simulink model "NewOrbitSimulation"  (R2015a)
settings: Solver=ode45  StartTime=0.0  StopTime=1000  FixedStep=.1  RelTol=1e-9
InitFcn:
  | PlanetSelect;
StopFcn:
  | TotalDeltaV
undefined symbols (not defined in the file or in its folder): AtmoAlt_planet, AtmoData, Cd, CraftInitialP, CraftInitialV, DragData, g0, GM_planet, GndAlt_planet, LastStage, Omega_planet, PitchOverAlt, PitchOverAngle, PitchSwitch, R_planet, RefSurfArea, SSIGN, TargetOrbit, Throttle
libraries: simulink_extras x6, dspmathops x5, simulink x3, vrlib x2
settings Model: PauseTimes=122  SnapshotInterval=1  Creator=raulm_000  LastModifiedBy=raulm_000
settings DataIOCC: ExternalInput=[Throttle,SSIGN]  LimitDataPoints=off  SaveFinalState=on

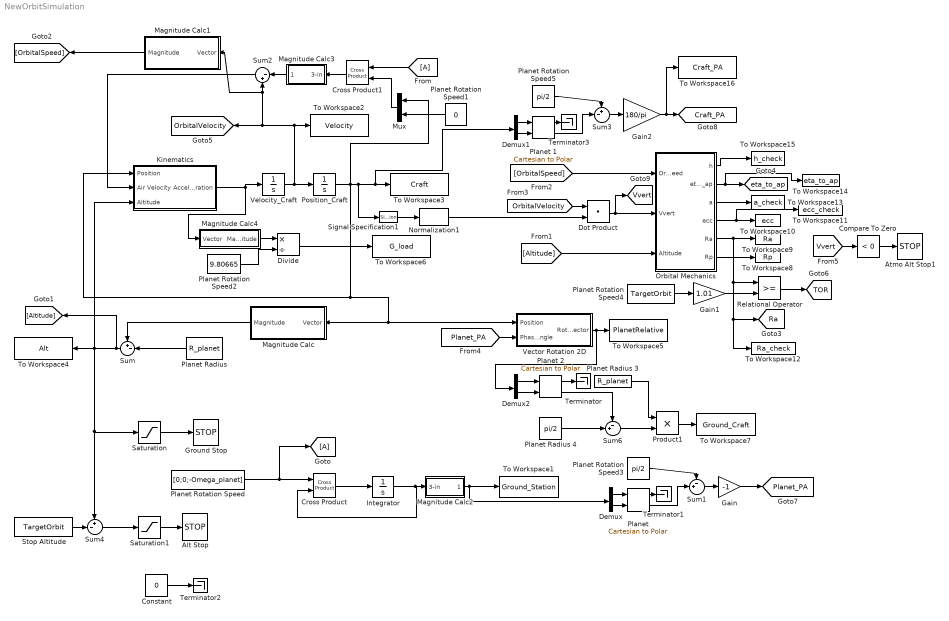
== system NewOrbitSimulation ==
  " Alt Stop" : Stop
  Atmo Alt Stop1 : Stop
  Compare To Zero : simulink/Logic and Bit Operations/Compare To Zero  relop=<  OutDataTypeStr=boolean
  Constant : Constant  Value=0
  Cross Product : vrlib/Utilities/Cross Product
  Cross Product1 : vrlib/Utilities/Cross Product
  Demux : Demux  Outputs=2
  Demux1 : Demux  Outputs=2
  Demux2 : Demux  Outputs=2
  Divide : Product  Inputs=*/
  Dot Product : DotProduct  InputSameDT=on  OutDataTypeStr=Inherit: Inherit via internal rule
  Gain : Gain  Gain=-1
  Gain1 : Gain  Gain=1.01
  Gain2 : Gain  Gain=180/pi
  Ground Stop : Stop
  Integrator : Integrator  InitialCondition=[0;R_planet;0]
  Kinematics : Subsystem
  Magnitude Calc : Subsystem
  Magnitude Calc1 : Subsystem
  Magnitude Calc2 : Subsystem
  Magnitude Calc3 : Subsystem
  Magnitude Calc4 : Subsystem
  Mux : Mux  Inputs=2
  Normalization1 : dspmathops/Normalization  NormType=2-norm  Bias=1e-10  NormOver=Specified dimension  ColComp=off  Dimension=1  outputMin=[]  outputMax=[]  accumDataTypeStr=Inherit: Same as product output  accumLastDataTypeStr=Inherit: Same as product output  roundingMode=Floor  overflowMode=off
  Orbital Mechanics : MATLAB Function  TreatAsAtomicUnit=on
  "Planet " : simulink_extras/Transformations/Cartesian to Polar
  Planet 1 : simulink_extras/Transformations/Cartesian to Polar
  Planet 2 : simulink_extras/Transformations/Cartesian to Polar
  "Planet Radius " : Constant  Value=R_planet
  Planet Radius 3 : Constant  Value=R_planet
  Planet Radius 4 : Constant  Value=pi/2
  Planet Rotation Speed : Constant  Value=[0;0;-Omega_planet]
  Planet Rotation Speed1 : Constant  Value=0
  Planet Rotation Speed2 : Constant  Value=9.80665
  Planet Rotation Speed3 : Constant  Value=pi/2
  Planet Rotation Speed4 : Constant  Value=TargetOrbit
  Planet Rotation Speed5 : Constant  Value=pi/2
  Position_Craft : Integrator  InitialCondition=CraftInitialP
  Product1 : Product
  Relational Operator : RelationalOperator  OutDataTypeStr=boolean
  Saturation : Saturate  UpperLimit=0
  Saturation1 : Saturate  UpperLimit=1  LowerLimit=0
  Signal Specification1 : SignalSpecification  Dimensions=2
  Stop Altitude : Constant  Value=TargetOrbit
  Sum : Sum  Inputs=+-|
  Sum1 : Sum  Inputs=-+|
  Sum2 : Sum  Inputs=|-+
  Sum3 : Sum  Inputs=+-|
  Sum4 : Sum  Inputs=+-|
  Sum6 : Sum  Inputs=-+|
  Terminator{,1..3} (4 alike) : Terminator
  To Workspace1 : ToWorkspace  VariableName=Ground_Station  SampleTime=-1
  To Workspace10 : ToWorkspace  VariableName=ecc  SampleTime=-1
  To Workspace11 : ToWorkspace  VariableName=ecc_check  SampleTime=-1
      settings: MaxDataPoints=1
  To Workspace12 : ToWorkspace  VariableName=Ra_check  SampleTime=-1
      settings: MaxDataPoints=1
  To Workspace13 : ToWorkspace  VariableName=a_check  SampleTime=-1
      settings: MaxDataPoints=1
  To Workspace14 : ToWorkspace  VariableName=eta_to_ap  SampleTime=-1
  To Workspace15 : ToWorkspace  VariableName=h_check  SampleTime=-1
      settings: MaxDataPoints=1
  To Workspace16 : ToWorkspace  VariableName=Craft_PA  SampleTime=-1
  To Workspace2 : ToWorkspace  VariableName=Velocity  SampleTime=-1
  To Workspace3 : ToWorkspace  VariableName=Craft  SampleTime=-1
  To Workspace4 : ToWorkspace  VariableName=Alt  SampleTime=-1
  To Workspace5 : ToWorkspace  VariableName=PlanetRelative  SampleTime=-1
  To Workspace6 : ToWorkspace  VariableName=G_load  SampleTime=-1
  To Workspace7 : ToWorkspace  VariableName=Ground_Craft  SampleTime=-1
  To Workspace8 : ToWorkspace  VariableName=Rp  SampleTime=-1
  To Workspace9 : ToWorkspace  VariableName=Ra  SampleTime=-1
  Vector Rotation 2D : Subsystem
  Velocity_Craft : Integrator  InitialCondition=CraftInitialV-[.1;0]
  tag scope: Craft_PA=global, OrbitalVelocity=global, Planet_PA=global, Ra=global, TOR=global, Vvert=global, eta_to_ap=global
  wires:
  Planet Rotation Speed/1 -> [A], Cross Product/1
  Integrator/1 -> Cross Product/2, Magnitude Calc2/1(3-in)
  Cross Product/1 -> Integrator/1
  Velocity_Craft/1 -> Position_Craft/1, [OrbitalVelocity], Magnitude Calc1/1(Vector), Sum2/2, To Workspace2/1
  Position_Craft/1 -> Mux/1, Kinematics/1(Position), Vector Rotation 2D/1(Position), Magnitude Calc/1(Vector), Signal Specification1/1, Demux1/1, To Workspace3/1
  Magnitude Calc/1("Magnitude ") -> Sum/1
  "Planet Radius "/1 -> Sum/2
  Sum/1 -> [Altitude], Kinematics/3("Altitude "), Sum4/1, Saturation/1, To Workspace4/1
  Magnitude Calc2/1("2-out ") -> Demux/1, To Workspace1/1
  Sum2/1 -> Kinematics/2(Air Velocity)
  Kinematics/1("Acceleration ") -> Velocity_Craft/1, Magnitude Calc4/1(Vector)
  Saturation/1 -> Ground Stop/1
  [A] -> Cross Product1/1
  Cross Product1/1 -> Magnitude Calc3/1(3-in)
  Mux/1 -> Cross Product1/2
  Planet Rotation Speed1/1 -> Mux/2
  Magnitude Calc3/1("2-out ") -> Sum2/1
  Stop Altitude/1 -> Sum4/2
  Sum4/1 -> Saturation1/1
  Magnitude Calc4/1("Magnitude ") -> Divide/1
  Planet Rotation Speed2/1 -> Divide/2
  Divide/1 -> To Workspace6/1
  Demux/1 -> "Planet "/1
  Demux/2 -> "Planet "/2
  Vector Rotation 2D/1("Rotated Vector ") -> Demux2/1, To Workspace5/1
  "Planet "/2 -> Sum1/2
  Planet Rotation Speed3/1 -> Sum1/1
  Sum1/1 -> Gain/1
  Planet 2/2 -> Sum6/1
  Planet Radius 3/1 -> Product1/1
  Product1/1 -> To Workspace7/1
  Planet Radius 4/1 -> Sum6/2
  Sum6/1 -> Product1/2
  Demux2/1 -> Planet 2/1
  Demux2/2 -> Planet 2/2
  Orbital Mechanics/5(Ra) -> To Workspace12/1, [Ra], Relational Operator/1, To Workspace9/1
  Orbital Mechanics/6(Rp) -> To Workspace8/1
  Orbital Mechanics/4(ecc) -> To Workspace11/1, To Workspace10/1
  Planet Rotation Speed4/1 -> Gain1/1
  Magnitude Calc1/1("Magnitude ") -> [OrbitalSpeed]
  [Altitude] -> Orbital Mechanics/3(Altitude)
  [OrbitalSpeed] -> Orbital Mechanics/1(OrbitalSpeed)
  Relational Operator/1 -> [TOR]
  Planet 2/1 -> Terminator/1
  "Planet "/1 -> Terminator1/1
  Orbital Mechanics/3(a) -> To Workspace13/1
  Orbital Mechanics/2(eta_to_ap) -> To Workspace14/1, [eta_to_ap]
  Orbital Mechanics/1(h) -> To Workspace15/1
  Signal Specification1/1 -> Normalization1/1
  Normalization1/1 -> Dot Product/2
  [OrbitalVelocity] -> Dot Product/1
  Dot Product/1 -> Orbital Mechanics/2(Vvert), [Vvert]
  Gain/1 -> [Planet_PA]
  [Planet_PA] -> Vector Rotation 2D/2(Phase Angle)
  Demux1/1 -> Planet 1/1
  Demux1/2 -> Planet 1/2
  Planet 1/2 -> Sum3/2
  Planet Rotation Speed5/1 -> Sum3/1
  Planet 1/1 -> Terminator3/1
  Constant/1 -> Terminator2/1
  Saturation1/1 -> " Alt Stop"/1
  Gain1/1 -> Relational Operator/2
  [Vvert] -> Compare To Zero/1
  Compare To Zero/1 -> Atmo Alt Stop1/1
  Sum3/1 -> Gain2/1
  Gain2/1 -> To Workspace16/1, [Craft_PA]

== system NewOrbitSimulation/Kinematics ==
  Position : Inport
  Air Velocity : Inport  Port=2
  "Altitude " : Inport  Port=3
  Aerodynamics : Subsystem
  Gravitational Acceleration : Subsystem
  Sum3 : Sum  Inputs=+++
  Thrust : Subsystem
  "Acceleration " : Outport
  wires:
  Position/1 -> Thrust/2(Position), Gravitational Acceleration/1(Position)
  Air Velocity/1 -> Thrust/3(AirVelocity), Aerodynamics/1(Air Velocity)
  "Altitude "/1 -> Thrust/1(Altitude), Aerodynamics/2("Altitude ")
  Aerodynamics/1("Aeroaccel ") -> Sum3/2
  Gravitational Acceleration/1("Gavity ") -> Sum3/1
  Sum3/1 -> "Acceleration "/1
  Thrust/1("ThrustAccel ") -> Sum3/3

== system NewOrbitSimulation/Magnitude Calc ==
  Vector : Inport
  Add : Sum
  Demux : Demux  Outputs=2
  Math Function : Math  Operator=square  SaturateOnIntegerOverflow=on
  Math Function1 : Math  Operator=square  SaturateOnIntegerOverflow=on
  Sqrt : Sqrt  SaturateOnIntegerOverflow=on
  "Magnitude " : Outport
  wires:
  Demux/1 -> Math Function1/1
  Demux/2 -> Math Function/1
  Math Function/1 -> Add/2
  Add/1 -> Sqrt/1
  Vector/1 -> Demux/1
  Math Function1/1 -> Add/1
  Sqrt/1 -> "Magnitude "/1

== system NewOrbitSimulation/Magnitude Calc1 ==
  Vector : Inport
  Add : Sum
  Demux : Demux  Outputs=2
  Math Function : Math  Operator=square  SaturateOnIntegerOverflow=on
  Math Function1 : Math  Operator=square  SaturateOnIntegerOverflow=on
  Sqrt : Sqrt  SaturateOnIntegerOverflow=on
  "Magnitude " : Outport
  wires:
  Demux/1 -> Math Function1/1
  Demux/2 -> Math Function/1
  Math Function/1 -> Add/2
  Add/1 -> Sqrt/1
  Vector/1 -> Demux/1
  Math Function1/1 -> Add/1
  Sqrt/1 -> "Magnitude "/1

== system NewOrbitSimulation/Magnitude Calc2 ==
  3-in : Inport
  Demux4 : Demux  Outputs=3
  Mux2 : Mux  Inputs=2
  Terminator3 : Terminator
  "2-out " : Outport
  wires:
  3-in/1 -> Demux4/1
  Demux4/3 -> Terminator3/1
  Demux4/1 -> Mux2/1
  Demux4/2 -> Mux2/2
  Mux2/1 -> "2-out "/1

== system NewOrbitSimulation/Magnitude Calc3 ==
  3-in : Inport
  Demux4 : Demux  Outputs=3
  Mux2 : Mux  Inputs=2
  Terminator3 : Terminator
  "2-out " : Outport
  wires:
  3-in/1 -> Demux4/1
  Demux4/3 -> Terminator3/1
  Demux4/1 -> Mux2/1
  Demux4/2 -> Mux2/2
  Mux2/1 -> "2-out "/1

== system NewOrbitSimulation/Magnitude Calc4 ==
  Vector : Inport
  Add : Sum
  Demux : Demux  Outputs=2
  Math Function : Math  Operator=square  SaturateOnIntegerOverflow=on
  Math Function1 : Math  Operator=square  SaturateOnIntegerOverflow=on
  Sqrt : Sqrt  SaturateOnIntegerOverflow=on
  "Magnitude " : Outport
  wires:
  Demux/1 -> Math Function1/1
  Demux/2 -> Math Function/1
  Math Function/1 -> Add/2
  Add/1 -> Sqrt/1
  Vector/1 -> Demux/1
  Math Function1/1 -> Add/1
  Sqrt/1 -> "Magnitude "/1

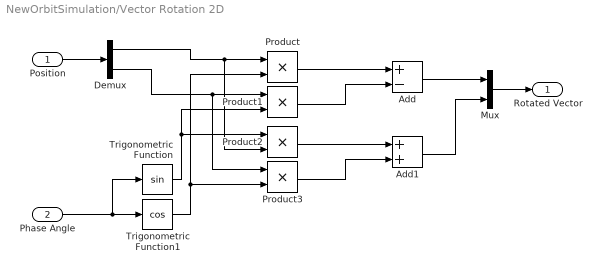
== system NewOrbitSimulation/Vector Rotation 2D ==
  Position : Inport
  Phase Angle : Inport  Port=2
  Add : Sum  Inputs=+-
  Add1 : Sum
  Demux : Demux  Outputs=2
  Mux : Mux  Inputs=2
  Product{,1..3} (4 alike) : Product
  Trigonometric Function : Trigonometry
  Trigonometric Function1 : Trigonometry  Operator=cos
  "Rotated Vector " : Outport
  wires:
  Mux/1 -> "Rotated Vector "/1
  Phase Angle/1 -> Trigonometric Function/1, Trigonometric Function1/1
  Position/1 -> Demux/1
  Trigonometric Function1/1 -> Product3/2, Product/2
  Demux/1 -> Product2/2, Product/1
  Product/1 -> Add/1
  Demux/2 -> Product3/1, Product1/1
  Trigonometric Function/1 -> Product2/1, Product1/2
  Product1/1 -> Add/2
  Product2/1 -> Add1/1
  Product3/1 -> Add1/2
  Add1/1 -> Mux/2
  Add/1 -> Mux/1

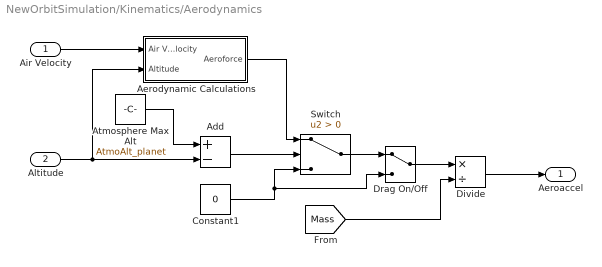
== system NewOrbitSimulation/Kinematics/Aerodynamics ==
  Air Velocity : Inport
  "Altitude " : Inport  Port=2
  Add : Sum  Inputs=+-
  Aerodynamic Calculations : Subsystem
  Atmosphere Max Alt : Constant  Value=AtmoAlt_planet
  Constant1 : Constant  Value=0
  Divide : Product  Inputs=*/
  Drag On/Off : ManualSwitch
  Switch : Switch  Criteria=u2 > Threshold
  "Aeroaccel " : Outport
  wires:
  "Altitude "/1 -> Aerodynamic Calculations/2(Altitude), Add/2
  Atmosphere Max Alt/1 -> Add/1
  Add/1 -> Switch/2
  Constant1/1 -> Drag On/Off/2, Switch/3
  Switch/1 -> Drag On/Off/1
  Drag On/Off/1 -> Divide/1
  Divide/1 -> "Aeroaccel "/1
  [Mass] -> Divide/2
  Air Velocity/1 -> Aerodynamic Calculations/1(Air Velocity)
  Aerodynamic Calculations/1("Aeroforce ") -> Switch/1

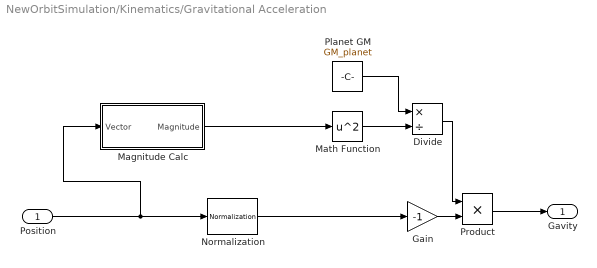
== system NewOrbitSimulation/Kinematics/Gravitational Acceleration ==
  Position : Inport
  Divide : Product  Inputs=*/
  Gain : Gain  Gain=-1
  Magnitude Calc : Subsystem
  Math Function : Math  Operator=square  SaturateOnIntegerOverflow=on
  Normalization : dspmathops/Normalization  NormType=2-norm  Bias=1e-10  NormOver=Specified dimension  ColComp=off  Dimension=1  outputDataTypeStr=Inherit: Same as product output  outputLastDataTypeStr=Inherit: Same as product output  outputMin=[]  outputMax=[]  accumDataTypeStr=Inherit: Same as product output  accumLastDataTypeStr=Inherit: Same as product output  roundingMode=Floor  overflowMode=off
  Planet GM : Constant  Value=GM_planet
  Product : Product
  "Gavity " : Outport
  wires:
  Position/1 -> Normalization/1, Magnitude Calc/1(Vector)
  Magnitude Calc/1("Magnitude ") -> Math Function/1
  Planet GM/1 -> Divide/1
  Math Function/1 -> Divide/2
  Product/1 -> "Gavity "/1
  Gain/1 -> Product/2
  Divide/1 -> Product/1
  Normalization/1 -> Gain/1

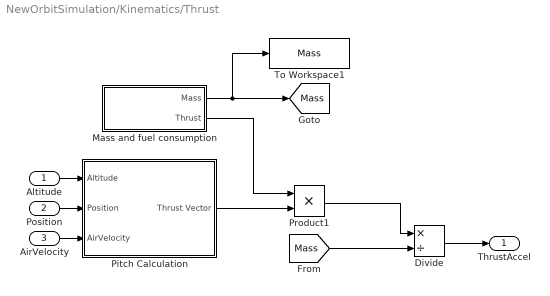
== system NewOrbitSimulation/Kinematics/Thrust ==
  Altitude : Inport
  Position : Inport  Port=2
  AirVelocity : Inport  Port=3
  Divide : Product  Inputs=*/
  Mass and fuel consumption : Subsystem
  Pitch Calculation : Subsystem
  Product1 : Product
  To Workspace1 : ToWorkspace  VariableName=Mass  SampleTime=-1
  "ThrustAccel " : Outport
  tag scope: Mass=global
  wires:
  Product1/1 -> Divide/1
  Mass and fuel consumption/1("Mass ") -> To Workspace1/1, [Mass]
  [Mass] -> Divide/2
  Mass and fuel consumption/2("Thrust ") -> Product1/1
  Position/1 -> Pitch Calculation/2(Position)
  Pitch Calculation/1(Thrust Vector) -> Product1/2
  Altitude/1 -> Pitch Calculation/1(Altitude)
  AirVelocity/1 -> Pitch Calculation/3(AirVelocity)
  Divide/1 -> "ThrustAccel "/1

== system NewOrbitSimulation/Kinematics/Aerodynamics/Aerodynamic Calculations ==
  Air Velocity : Inport
  Altitude : Inport  Port=2
  Cl and Cd Calculation : Subsystem
  Magnitude Calc1 : Subsystem
  Product : Product  Inputs=3
  Referance Surface Area : Constant  Value=RefSurfArea
  "Aeroforce " : Outport
  wires:
  Air Velocity/1 -> Cl and Cd Calculation/1(Airspeed), Magnitude Calc1/1(Air Velocity)
  Referance Surface Area/1 -> Product/2
  Altitude/1 -> Magnitude Calc1/2("Altitude "), Cl and Cd Calculation/2("Altitude ")
  Cl and Cd Calculation/1(Cl + Cd) -> Product/3
  Product/1 -> "Aeroforce "/1
  Magnitude Calc1/1("Dynamic Pressure ") -> Product/1

== system NewOrbitSimulation/Kinematics/Gravitational Acceleration/Magnitude Calc ==
  Vector : Inport
  Add : Sum
  Demux : Demux  Outputs=2
  Math Function : Math  Operator=square  SaturateOnIntegerOverflow=on
  Math Function1 : Math  Operator=square  SaturateOnIntegerOverflow=on
  Sqrt : Sqrt  SaturateOnIntegerOverflow=on
  "Magnitude " : Outport
  wires:
  Demux/1 -> Math Function1/1
  Demux/2 -> Math Function/1
  Math Function/1 -> Add/2
  Add/1 -> Sqrt/1
  Vector/1 -> Demux/1
  Math Function1/1 -> Add/1
  Sqrt/1 -> "Magnitude "/1

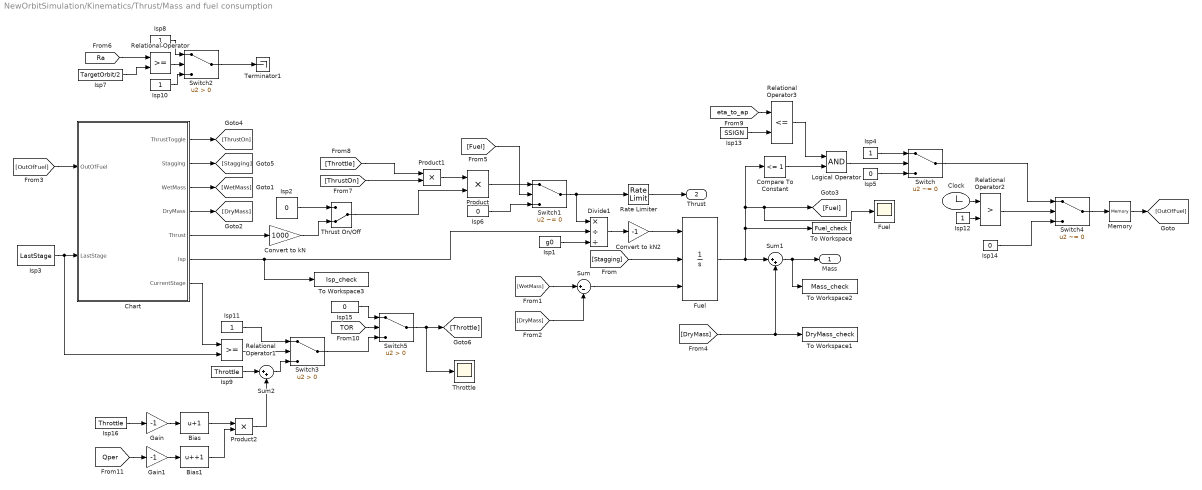
== system NewOrbitSimulation/Kinematics/Thrust/Mass and fuel consumption ==
  Bias : Bias  Bias=1
  Bias1 : Bias  Bias=+1
  Chart : Stateflow chart  TreatAsAtomicUnit=on
  Clock : Clock
  Compare To Constant : simulink/Logic and Bit Operations/Compare To Constant  relop=<=  const=1  OutDataTypeStr=boolean
  Convert to kN : Gain  Gain=1000
  Convert to kN2 : Gain  Gain=-1
  Divide1 : Product  Inputs=*//
  Fuel : Integrator  ExternalReset=rising  InitialConditionSource=external  LimitOutput=on  LowerSaturationLimit=0
  "Fuel " : Scope
      settings: SaveName=ScopeData4
  Gain : Gain  Gain=-1
  Gain1 : Gain  Gain=-1
  Isp1 : Constant  Value=g0
  Isp{4,8,10..12} (5 alike) : Constant
  Isp13 : Constant  Value=SSIGN
  Isp{2,5..6,14..15} (5 alike) : Constant  Value=0
  Isp16 : Constant  Value=Throttle
  Isp3 : Constant  Value=LastStage
  Isp7 : Constant  Value=TargetOrbit/2
  Isp9 : Constant  Value=Throttle
  Logical Operator : Logic  AllPortsSameDT=off  OutDataTypeStr=boolean
  Memory : Memory
  Product : Product
  Product1 : Product
  Product2 : Product
  Rate Limiter : RateLimiter  RisingSlewLimit=100000  FallingSlewLimit=-100000  SampleTimeMode=inherited
  Relational Operator : RelationalOperator  OutDataTypeStr=boolean
  Relational Operator1 : RelationalOperator  OutDataTypeStr=boolean
  Relational Operator2 : RelationalOperator  Operator=>  OutDataTypeStr=boolean
  Relational Operator3 : RelationalOperator  Operator=<=  OutDataTypeStr=boolean
  Sum : Sum  Inputs=|+-
  Sum1 : Sum  Inputs=|++
  Sum2 : Sum  Inputs=|++
  Switch : Switch  Criteria=u2 ~= 0
  Switch1 : Switch  Criteria=u2 ~= 0
  Switch2 : Switch  Criteria=u2 > Threshold
  Switch3 : Switch  Criteria=u2 > Threshold
  Switch4 : Switch  Criteria=u2 ~= 0
  Switch5 : Switch  Criteria=u2 > Threshold
  Terminator1 : Terminator
  Throttle : Scope
  Thrust On/Off : ManualSwitch  CurrentSetting=0
  To Workspace : ToWorkspace  VariableName=Fuel_check  SampleTime=-1
      settings: MaxDataPoints=1
  To Workspace1 : ToWorkspace  VariableName=DryMass_check  SampleTime=-1
      settings: MaxDataPoints=1
  To Workspace2 : ToWorkspace  VariableName=Mass_check  SampleTime=-1
      settings: MaxDataPoints=1
  To Workspace3 : ToWorkspace  VariableName=Isp_check  SampleTime=-1
      settings: MaxDataPoints=1
  "Mass " : Outport
  "Thrust " : Outport  Port=2
  wires:
  Isp1/1 -> Divide1/3
  Divide1/1 -> Convert to kN2/1
  Convert to kN2/1 -> Fuel/1
  Isp2/1 -> Thrust On/Off/1
  Convert to kN/1 -> Thrust On/Off/2
  Sum/1 -> Fuel/3
  Sum1/1 -> To Workspace2/1, "Mass "/1
  [WetMass] -> Sum/1
  [DryMass] -> Sum/2
  [DryMass] -> Sum1/2, To Workspace1/1
  [OutOfFuel] -> Chart/1(OutOfFuel)
  Isp3/1 -> Relational Operator1/2, Chart/2(LastStage)
  Thrust On/Off/1 -> Product/2
  Chart/2(Stagging) -> [Stagging]
  [Stagging] -> Fuel/2
  Chart/3(WetMass) -> [WetMass]
  Chart/4(DryMass) -> [DryMass]
  Chart/5(Thrust) -> Convert to kN/1
  Chart/6(Isp) -> To Workspace3/1, Divide1/2
  Isp4/1 -> Switch/1
  Isp5/1 -> Switch/3
  Switch1/1 -> Rate Limiter/1, Divide1/1
  Product/1 -> Switch1/1
  Isp7/1 -> Relational Operator/2
  [Ra] -> Relational Operator/1
  Relational Operator/1 -> Switch2/2
  [ThrustOn] -> Product1/2
  Product1/1 -> Product/1
  Isp10/1 -> Switch2/3
  Isp8/1 -> Switch2/1
  Rate Limiter/1 -> "Thrust "/1
  [Fuel] -> Switch1/2
  Isp6/1 -> Switch1/3
  Chart/1(ThrustToggle) -> [ThrustOn]
  Chart/7(CurrentStage) -> Relational Operator1/1
  Relational Operator1/1 -> Switch3/2
  Isp11/1 -> Switch3/1
  [Throttle] -> Product1/1
  Switch2/1 -> Terminator1/1
  [eta_to_ap] -> Relational Operator3/1
  Isp13/1 -> Relational Operator3/2
  Relational Operator3/1 -> Logical Operator/1
  Fuel/1 -> Compare To Constant/1, "Fuel "/1, [Fuel], To Workspace/1, Sum1/1
  Clock/1 -> Relational Operator2/1
  Isp12/1 -> Relational Operator2/2
  Relational Operator2/1 -> Switch4/2
  Switch/1 -> Switch4/1
  Isp14/1 -> Switch4/3
  Switch4/1 -> Memory/1
  Memory/1 -> [OutOfFuel]
  Compare To Constant/1 -> Logical Operator/2
  Logical Operator/1 -> Switch/2
  [TOR] -> Switch5/2
  Switch3/1 -> Switch5/3
  Switch5/1 -> Throttle/1, [Throttle]
  Isp15/1 -> Switch5/1
  Isp16/1 -> Gain/1
  Gain/1 -> Bias/1
  Bias/1 -> Product2/1
  Bias1/1 -> Product2/2
  Isp9/1 -> Sum2/1
  Product2/1 -> Sum2/2
  Sum2/1 -> Switch3/3
  [Qper] -> Gain1/1
  Gain1/1 -> Bias1/1

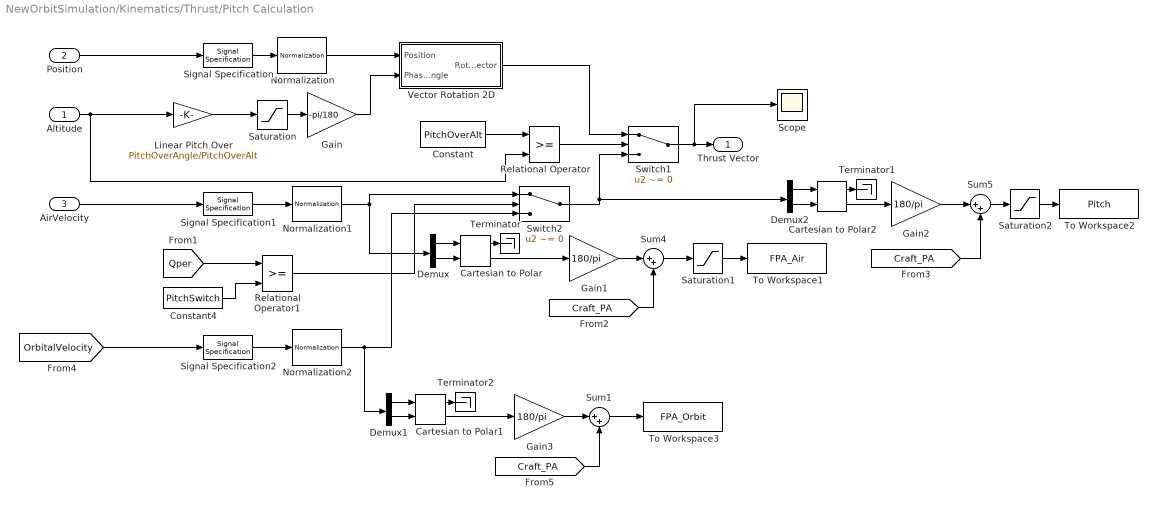
== system NewOrbitSimulation/Kinematics/Thrust/Pitch Calculation ==
  Altitude : Inport  PortDimensions=1
  Position : Inport  Port=2
  AirVelocity : Inport  Port=3
  Cartesian to Polar : simulink_extras/Transformations/Cartesian to Polar
  Cartesian to Polar1 : simulink_extras/Transformations/Cartesian to Polar
  Cartesian to Polar2 : simulink_extras/Transformations/Cartesian to Polar
  Constant : Constant  Value=PitchOverAlt
  Constant4 : Constant  Value=PitchSwitch
  Demux : Demux  Outputs=2
  Demux1 : Demux  Outputs=2
  Demux2 : Demux  Outputs=2
  Gain : Gain  Gain=-pi/180
  Gain1 : Gain  Gain=180/pi
  Gain2 : Gain  Gain=180/pi
  Gain3 : Gain  Gain=180/pi
  Linear Pitch Over : Gain  Gain=PitchOverAngle/PitchOverAlt
  Normalization : dspmathops/Normalization  NormType=2-norm  Bias=1e-10  NormOver=Specified dimension  ColComp=off  Dimension=1  outputMin=[]  outputMax=[]  accumDataTypeStr=Inherit: Same as product output  accumLastDataTypeStr=Inherit: Same as product output  roundingMode=Floor  overflowMode=off
  Normalization1 : dspmathops/Normalization  NormType=2-norm  Bias=1e-10  NormOver=Specified dimension  ColComp=off  Dimension=1  outputMin=[]  outputMax=[]  accumDataTypeStr=Inherit: Same as product output  accumLastDataTypeStr=Inherit: Same as product output  roundingMode=Floor  overflowMode=off
  Normalization2 : dspmathops/Normalization  NormType=2-norm  Bias=1e-10  NormOver=Specified dimension  ColComp=off  Dimension=1  outputMin=[]  outputMax=[]  accumDataTypeStr=Inherit: Same as product output  accumLastDataTypeStr=Inherit: Same as product output  roundingMode=Floor  overflowMode=off
  Relational Operator : RelationalOperator  OutDataTypeStr=boolean
  Relational Operator1 : RelationalOperator  OutDataTypeStr=boolean
  Saturation : Saturate  UpperLimit=90  LowerLimit=0
  Saturation1 : Saturate  UpperLimit=90  LowerLimit=0
  Saturation2 : Saturate  UpperLimit=90  LowerLimit=0
  Scope : Scope
  Signal Specification : SignalSpecification  Dimensions=2
  Signal Specification1 : SignalSpecification  Dimensions=2
  Signal Specification2 : SignalSpecification  Dimensions=2
  Sum1 : Sum  Inputs=|++
  Sum4 : Sum  Inputs=|++
  Sum5 : Sum  Inputs=|++
  Switch1 : Switch  Criteria=u2 ~= 0  Threshold=PitchOverAlt
  Switch2 : Switch  Criteria=u2 ~= 0  Threshold=PitchOverAlt
  Terminator : Terminator
  Terminator1 : Terminator
  Terminator2 : Terminator
  To Workspace1 : ToWorkspace  VariableName=FPA_Air  SampleTime=-1
  To Workspace2 : ToWorkspace  VariableName=Pitch  SampleTime=-1
  To Workspace3 : ToWorkspace  VariableName=FPA_Orbit  SampleTime=-1
  Vector Rotation 2D : Subsystem
  Thrust Vector : Outport
  wires:
  Position/1 -> Signal Specification/1
  Signal Specification/1 -> Normalization/1
  AirVelocity/1 -> Signal Specification1/1
  Signal Specification1/1 -> Normalization1/1
  Normalization/1 -> Vector Rotation 2D/1(Position)
  Relational Operator/1 -> Switch1/2
  Normalization1/1 -> Switch2/1, Demux/1
  Constant/1 -> Relational Operator/1
  Demux/1 -> Cartesian to Polar/1
  Demux/2 -> Cartesian to Polar/2
  Vector Rotation 2D/1("Rotated Vector ") -> Switch1/1
  Linear Pitch Over/1 -> Saturation/1
  Saturation/1 -> Gain/1
  Gain/1 -> Vector Rotation 2D/2(Phase Angle)
  Altitude/1 -> Linear Pitch Over/1, Relational Operator/2
  Switch1/1 -> Scope/1, Thrust Vector/1
  Cartesian to Polar/1 -> Terminator/1
  Signal Specification2/1 -> Normalization2/1
  [OrbitalVelocity] -> Signal Specification2/1
  Normalization2/1 -> Switch2/3, Demux1/1
  Demux1/1 -> Cartesian to Polar1/1
  Demux1/2 -> Cartesian to Polar1/2
  Sum1/1 -> To Workspace3/1
  Cartesian to Polar1/1 -> Terminator2/1
  [Qper] -> Relational Operator1/1
  Constant4/1 -> Relational Operator1/2
  Relational Operator1/1 -> Switch2/2
  Switch2/1 -> Demux2/1, Switch1/3
  Cartesian to Polar/2 -> Gain1/1
  Demux2/1 -> Cartesian to Polar2/1
  Demux2/2 -> Cartesian to Polar2/2
  Cartesian to Polar2/1 -> Terminator1/1
  Cartesian to Polar2/2 -> Gain2/1
  [Craft_PA] -> Sum5/2
  Gain2/1 -> Sum5/1
  Gain1/1 -> Sum4/1
  [Craft_PA] -> Sum4/2
  [Craft_PA] -> Sum1/2
  Gain3/1 -> Sum1/1
  Cartesian to Polar1/2 -> Gain3/1
  Saturation1/1 -> To Workspace1/1
  Sum4/1 -> Saturation1/1
  Sum5/1 -> Saturation2/1
  Saturation2/1 -> To Workspace2/1

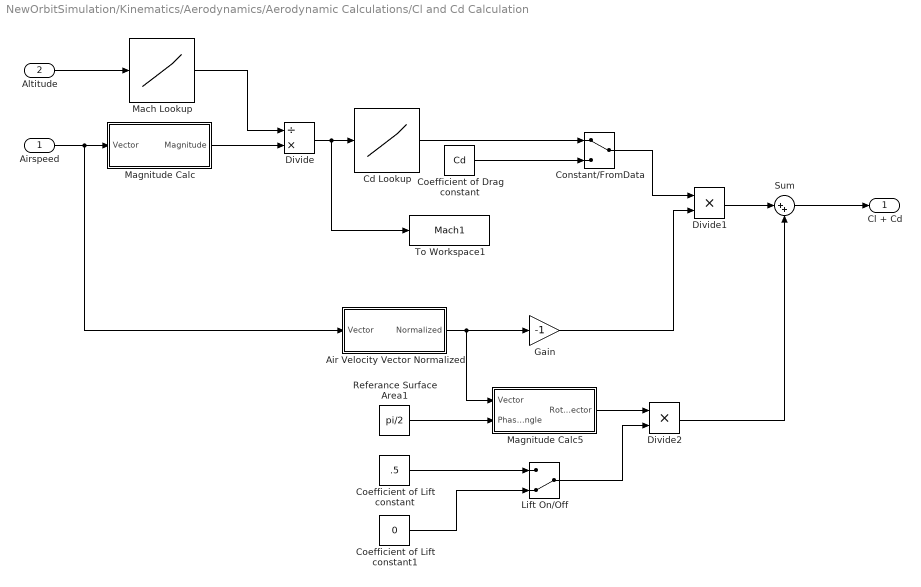
== system NewOrbitSimulation/Kinematics/Aerodynamics/Aerodynamic Calculations/Cl and Cd Calculation ==
  Airspeed : Inport
  "Altitude " : Inport  Port=2
  Air Velocity Vector Normalized : Subsystem
  Cd Lookup : Lookup_n-D  NumberOfTableDimensions=1  BreakpointsForDimension1=DragData(:,1)  Table=DragData(:,2)  InternalRulePriority=Speed  RndMeth=Simplest  InputSameDT=on
  Coefficient of Drag constant : Constant  Value=Cd
  Coefficient of Lift constant : Constant  Value=.5
  Coefficient of Lift constant1 : Constant  Value=0
  "Constant/FromData " : ManualSwitch
  Divide : Product  Inputs=/*
  Divide1 : Product  Inputs=**
  Divide2 : Product  Inputs=**
  Gain : Gain  Gain=-1
  Lift On/Off : ManualSwitch  CurrentSetting=0
  Mach Lookup : Lookup_n-D  NumberOfTableDimensions=1  BreakpointsForDimension1=AtmoData(:,1)  Table=AtmoData(:,4)  InternalRulePriority=Speed  RndMeth=Simplest  InputSameDT=on
  Magnitude Calc : Subsystem
  Magnitude Calc5 : Subsystem
  Referance Surface Area1 : Constant  Value=pi/2
  Sum : Sum  Inputs=|++
  To Workspace1 : ToWorkspace  VariableName=Mach1  SampleTime=-1
  Cl + Cd : Outport
  wires:
  "Altitude "/1 -> Mach Lookup/1
  Airspeed/1 -> Air Velocity Vector Normalized/1(Vector), Magnitude Calc/1(Vector)
  Magnitude Calc/1("Magnitude ") -> Divide/2
  Mach Lookup/1 -> Divide/1
  Divide/1 -> To Workspace1/1, Cd Lookup/1
  Cd Lookup/1 -> "Constant/FromData "/1
  Coefficient of Drag constant/1 -> "Constant/FromData "/2
  Air Velocity Vector Normalized/1("Normalized ") -> Magnitude Calc5/1(Vector), Gain/1
  Gain/1 -> Divide1/2
  "Constant/FromData "/1 -> Divide1/1
  Divide1/1 -> Sum/1
  Referance Surface Area1/1 -> Magnitude Calc5/2(Phase Angle)
  Magnitude Calc5/1("Rotated Vector ") -> Divide2/1
  Divide2/1 -> Sum/2
  Sum/1 -> Cl + Cd/1
  Coefficient of Lift constant1/1 -> Lift On/Off/2
  Coefficient of Lift constant/1 -> Lift On/Off/1
  Lift On/Off/1 -> Divide2/2

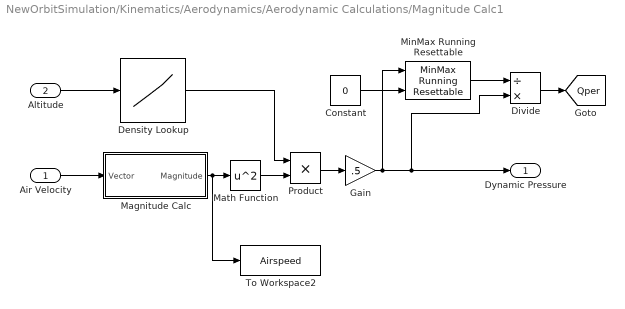
== system NewOrbitSimulation/Kinematics/Aerodynamics/Aerodynamic Calculations/Magnitude Calc1 ==
  Air Velocity : Inport
  "Altitude " : Inport  Port=2
  Constant : Constant  Value=0
  Density Lookup : Lookup_n-D  NumberOfTableDimensions=1  BreakpointsForDimension1=AtmoData(:,1)  Table=AtmoData(:,3)  InternalRulePriority=Speed  RndMeth=Simplest  InputSameDT=on
  Divide : Product  Inputs=/*
  Gain : Gain  Gain=.5
  Magnitude Calc : Subsystem
  Math Function : Math  Operator=square  SaturateOnIntegerOverflow=on
  MinMax Running Resettable : simulink/Math Operations/MinMax Running Resettable  Function=max  vinit=0.0
  Product : Product
  To Workspace2 : ToWorkspace  VariableName=Airspeed  SampleTime=-1
  "Dynamic Pressure " : Outport
  tag scope: Qper=global
  wires:
  "Altitude "/1 -> Density Lookup/1
  Magnitude Calc/1("Magnitude ") -> To Workspace2/1, Math Function/1
  Air Velocity/1 -> Magnitude Calc/1(Vector)
  Math Function/1 -> Product/2
  Product/1 -> Gain/1
  Density Lookup/1 -> Product/1
  MinMax Running Resettable/1 -> Divide/1
  Constant/1 -> MinMax Running Resettable/2
  Gain/1 -> MinMax Running Resettable/1, Divide/2, "Dynamic Pressure "/1
  Divide/1 -> [Qper]

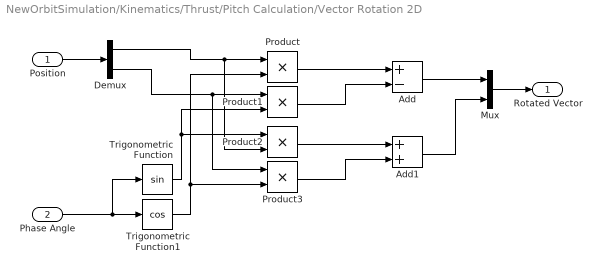
== system NewOrbitSimulation/Kinematics/Thrust/Pitch Calculation/Vector Rotation 2D ==
  Position : Inport
  Phase Angle : Inport  Port=2
  Add : Sum  Inputs=+-
  Add1 : Sum
  Demux : Demux  Outputs=2
  Mux : Mux  Inputs=2
  Product{,1..3} (4 alike) : Product
  Trigonometric Function : Trigonometry
  Trigonometric Function1 : Trigonometry  Operator=cos
  "Rotated Vector " : Outport
  wires:
  Mux/1 -> "Rotated Vector "/1
  Phase Angle/1 -> Trigonometric Function/1, Trigonometric Function1/1
  Position/1 -> Demux/1
  Trigonometric Function1/1 -> Product3/2, Product/2
  Demux/1 -> Product2/2, Product/1
  Product/1 -> Add/1
  Demux/2 -> Product3/1, Product1/1
  Trigonometric Function/1 -> Product2/1, Product1/2
  Product1/1 -> Add/2
  Product2/1 -> Add1/1
  Product3/1 -> Add1/2
  Add1/1 -> Mux/2
  Add/1 -> Mux/1

== system NewOrbitSimulation/Kinematics/Aerodynamics/Aerodynamic Calculations/Cl and Cd Calculation/Air Velocity Vector Normalized ==
  Vector : Inport
  Constant : Constant
  Demux3 : Demux  Outputs=2
  Divide1 : Product  Inputs=*/
  Divide2 : Product  Inputs=*/
  Magnitude Calc : Subsystem
  Mux1 : Mux  Inputs=2
  Switch : Switch  Criteria=u2 > Threshold
  "Normalized " : Outport
  wires:
  Demux3/1 -> Divide1/1
  Vector/1 -> Demux3/1, Magnitude Calc/1(Vector)
  Mux1/1 -> "Normalized "/1
  Demux3/2 -> Divide2/1
  Constant/1 -> Switch/3
  Magnitude Calc/1("Magnitude ") -> Switch/1
  Magnitude Calc/2(Is Zero) -> Switch/2
  Divide1/1 -> Mux1/1
  Divide2/1 -> Mux1/2
  Switch/1 -> Divide2/2, Divide1/2

== system NewOrbitSimulation/Kinematics/Aerodynamics/Aerodynamic Calculations/Cl and Cd Calculation/Magnitude Calc ==
  Vector : Inport
  Add : Sum
  Demux : Demux  Outputs=2
  Math Function : Math  Operator=square  SaturateOnIntegerOverflow=on
  Math Function1 : Math  Operator=square  SaturateOnIntegerOverflow=on
  Sqrt : Sqrt  SaturateOnIntegerOverflow=on
  "Magnitude " : Outport
  wires:
  Demux/1 -> Math Function1/1
  Demux/2 -> Math Function/1
  Math Function/1 -> Add/2
  Add/1 -> Sqrt/1
  Vector/1 -> Demux/1
  Math Function1/1 -> Add/1
  Sqrt/1 -> "Magnitude "/1

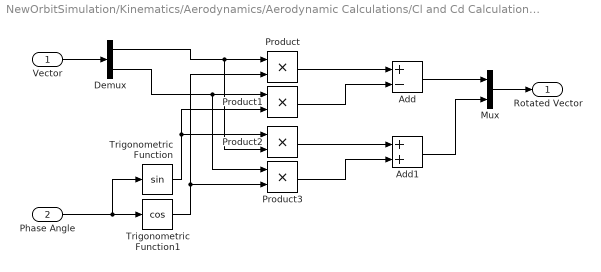
== system NewOrbitSimulation/Kinematics/Aerodynamics/Aerodynamic Calculations/Cl and Cd Calculation/Magnitude Calc5 ==
  Vector : Inport
  Phase Angle : Inport  Port=2
  Add : Sum  Inputs=+-
  Add1 : Sum
  Demux : Demux  Outputs=2
  Mux : Mux  Inputs=2
  Product{,1..3} (4 alike) : Product
  Trigonometric Function : Trigonometry
  Trigonometric Function1 : Trigonometry  Operator=cos
  "Rotated Vector " : Outport
  wires:
  Mux/1 -> "Rotated Vector "/1
  Phase Angle/1 -> Trigonometric Function/1, Trigonometric Function1/1
  Vector/1 -> Demux/1
  Trigonometric Function1/1 -> Product3/2, Product/2
  Demux/1 -> Product2/2, Product/1
  Product/1 -> Add/1
  Demux/2 -> Product3/1, Product1/1
  Trigonometric Function/1 -> Product2/1, Product1/2
  Product1/1 -> Add/2
  Product2/1 -> Add1/1
  Product3/1 -> Add1/2
  Add1/1 -> Mux/2
  Add/1 -> Mux/1

== system NewOrbitSimulation/Kinematics/Aerodynamics/Aerodynamic Calculations/Magnitude Calc1/Magnitude Calc ==
  Vector : Inport
  Add : Sum
  Demux : Demux  Outputs=2
  Math Function : Math  Operator=square  SaturateOnIntegerOverflow=on
  Math Function1 : Math  Operator=square  SaturateOnIntegerOverflow=on
  Sqrt : Sqrt  SaturateOnIntegerOverflow=on
  "Magnitude " : Outport
  wires:
  Demux/1 -> Math Function1/1
  Demux/2 -> Math Function/1
  Math Function/1 -> Add/2
  Add/1 -> Sqrt/1
  Vector/1 -> Demux/1
  Math Function1/1 -> Add/1
  Sqrt/1 -> "Magnitude "/1

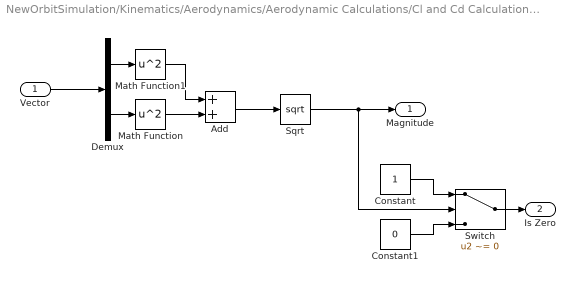
== system NewOrbitSimulation/Kinematics/Aerodynamics/Aerodynamic Calculations/Cl and Cd Calculation/Air Velocity Vector Normalized/Magnitude Calc ==
  Vector : Inport
  Add : Sum
  Constant : Constant
  Constant1 : Constant  Value=0
  Demux : Demux  Outputs=2
  Math Function : Math  Operator=square  SaturateOnIntegerOverflow=on
  Math Function1 : Math  Operator=square  SaturateOnIntegerOverflow=on
  Sqrt : Sqrt  SaturateOnIntegerOverflow=on
  Switch : Switch  Criteria=u2 ~= 0
  "Magnitude " : Outport
  Is Zero : Outport  Port=2
  wires:
  Demux/1 -> Math Function1/1
  Demux/2 -> Math Function/1
  Math Function/1 -> Add/2
  Add/1 -> Sqrt/1
  Vector/1 -> Demux/1
  Math Function1/1 -> Add/1
  Switch/1 -> Is Zero/1
  Constant/1 -> Switch/1
  Constant1/1 -> Switch/3
  Sqrt/1 -> Switch/2, "Magnitude "/1

== matlab function NewOrbitSimulation/Orbital Mechanics ==
  data: h output; eta_to_ap output; a output; OrbitalSpeed input; Vvert input; ecc output size=1; Altitude input; GM_planet parameter size=1; Ra output size=1; Rp output size=1; R_planet parameter; GndAlt_planet parameter
function [h,eta_to_ap,a,ecc,Ra,Rp] = fcn(OrbitalSpeed,Vvert,Altitude,GM_planet,R_planet,GndAlt_planet)
%#codegen
Radius = Altitude + R_planet;
Vpar = Vvert;
Vper = sqrt(abs(OrbitalSpeed^2 - Vpar^2));
h = Radius*Vper;

E = OrbitalSpeed^2/2 - GM_planet/Radius;
a = -GM_planet/(2*E);

ecc = sqrt(abs(1-((-2*E)*h^2)/(GM_planet^2)));

Ra = a*(1 + ecc) - (R_planet - GndAlt_planet);
Rp = a*(1 - ecc) - (R_planet - GndAlt_planet);

Theta = acosd(complex((1/ecc)*((h^2)/(GM_planet*Radius) - 1)));
%Theta = 0;
n = sqrt(abs(GM_planet/(a^3)));

EA = 2*atand(sqrt(abs(((1-ecc)/(1+ecc))*(tand(Theta/2)))));

MA = EA*pi/180 - ecc*sind(EA);
Delta_MA = pi - MA;

eta_to_ap = Delta_MA/n;

== stateflow chart NewOrbitSimulation/Kinematics/Thrust/Mass and fuel consumption/Chart ==
  settings: executeAtInitialization=1  initializeOutput=1
  state Start
    entry: Stage = 1;
  state Stage_Rocket_finish
    entry: ThrustToggle = 0
    entry: Stagging = 0
  state Nominal
    entry: ThrustToggle = 1;
    entry: Stagging = 0;
    entry: CurrentStage = Stage;
    entry: WetMass = ThrustMassData(Stage,1);
    entry: DryMass = ThrustMassData(Stage,2);
    entry: Thrust = ThrustMassData(Stage,3);
    entry: Isp = ThrustMassData(Stage,4);
  state Stage_Rocket
    entry: ThrustToggle = 0;
    entry: Stagging = 1;
    entry: Stage = Stage + 1;
    entry: WetMass = ThrustMassData(Stage,1);
    entry: DryMass = ThrustMassData(Stage,2);
    entry: Thrust = ThrustMassData(Stage,3);
    entry: Isp = ThrustMassData(Stage,4);
  (default) -> Start
  Start -> Nominal : [Stage == 1]
  Nominal -> Stage_Rocket_finish [order 2] : [OutOfFuel == 1 && Stage == LastStage]
  Nominal -> Stage_Rocket [order 1] : [OutOfFuel == 1 && Stage < LastStage]
  Stage_Rocket -> Nominal : [OutOfFuel == 0 && Stage <= LastStage]
  data: OutOfFuel input; ThrustToggle output; Stagging output; LastStage input; Stage local; WetMass output; DryMass output; Thrust output; Isp output; ThrustMassData parameter; CurrentStage output
